simulink model "labor13_Sim"  (R2024a)
settings: Solver=VariableStepAuto  StartTime=0.0  StopTime=100  MaxStep=0.1  RelTol=1e-3
values from neighbouring files (symbols this model uses):
  A = [0 1;-k/m -b/m]    [lab_13.m]    (also in labor13.m)
  Az = [A B;0 0 0]    [labor13.m]
  B = [0;1/m]    [lab_13.m]    (also in labor13.m)
  Bz = [B;0]    [labor13.m]
  C = [1 0]    [lab_13.m]    (also in labor13.m)
  Cz = [C 0]    [labor13.m]
  Gz = acker(Az',Cz',[so1 so2 so3])'    [labor13.m]
  K = acker(A,B,[sc1 sc2])    [lab_13.m]    (also in labor13.m)
  Mu = Mxu(end)    [lab_13.m]    (also in labor13.m)
  Mx = Mxu(1:2)    [lab_13.m]    (also in labor13.m)
libraries: simulink x1
settings Model: Creator=hallgato  LastModifiedBy=hallgato

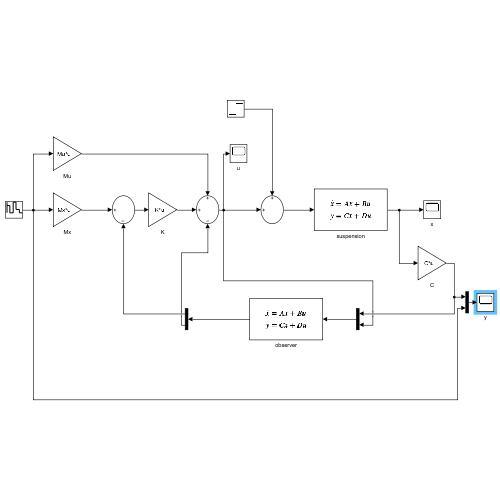
[thumbnail: Simulink's stored preview of the top-level diagram]
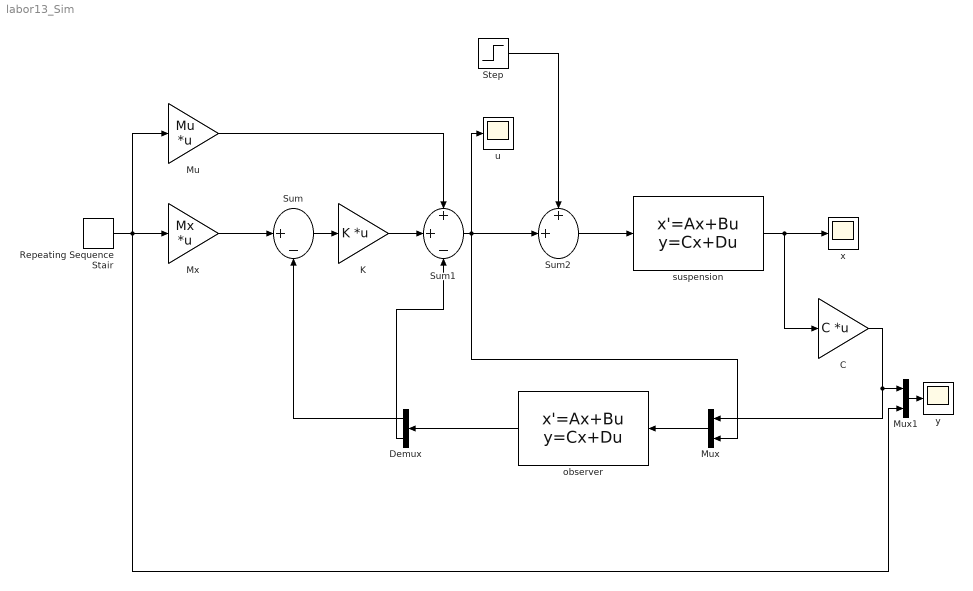
== system labor13_Sim ==
  C : Gain  Gain=C  Multiplication=Matrix(K*u)
  Demux : Demux  Outputs=2
  K : Gain  Gain=K  Multiplication=Matrix(K*u)
  Mu : Gain  Gain=Mu  Multiplication=Matrix(K*u)
  Mux : Mux  Inputs=2
  Mux1 : Mux  Inputs=2
  Mx : Gain  Gain=Mx  Multiplication=Matrix(K*u)
  Repeating Sequence Stair : simulink/Sources/Repeating Sequence Stair  OutValues=[3 1 4 2 1].'  tsamp=20  OutMin=[]  OutMax=[]  OutDataTypeStr=double  OutputDataTypeScalingMode=double  OutDataType=fixdt(0,8)  ConRadixGroup=Best Precision: Vector-wise  OutScaling=2^-12
  Step : Step  Time=20  After=10000  SampleTime=0
  Sum : Sum  Inputs=|+-
  Sum1 : Sum  Inputs=++-
  Sum2 : Sum  Inputs=++|
  observer : StateSpace  A=Az-Gz*Cz  B=[Gz Bz]  C=eye(3)  D=zeros(3,2)  InitialCondition=[0 0 0]
  suspension : StateSpace  A=A  B=B  C=eye(2)  D=zeros(2,1)  InitialCondition=[0.1 0]
  u : Scope
  x : Scope
  y : Scope
  wires:
  suspension/1 -> C/1, x/1
  Sum/1 -> K/1
  Mx/1 -> Sum/1
  Repeating Sequence Stair/1 -> Mux1/2, Mu/1, Mx/1
  K/1 -> Sum1/2
  Mu/1 -> Sum1/1
  C/1 -> Mux1/1, Mux/1
  Mux/1 -> observer/1
  Sum1/1 -> Mux/2, u/1, Sum2/2
  Sum2/1 -> suspension/1
  Step/1 -> Sum2/1
  Mux1/1 -> y/1
  observer/1 -> Demux/1
  Demux/1 -> Sum/2
  Demux/2 -> Sum1/3
